simulink model "vanderpol_simulink"  (R2013a)
settings: Solver=ode45  StartTime=0.0  StopTime=2  RelTol=1e-3
settings Model: Creator=zutshi  LastModifiedBy=zutshi

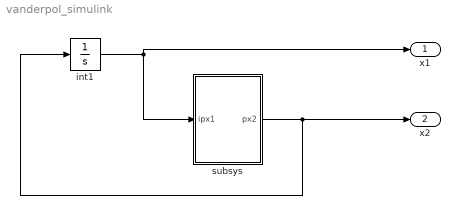
== system vanderpol_simulink ==
  int1 : Integrator  InitialCondition=0.4611  ContinuousStateAttributes='x1'
  subsys : Subsystem
  x1 : Outport
  x2 : Outport  Port=2
  wires:
  int1/1 -> x1/1, subsys/1(ipx1)
  subsys/1(px2) -> x2/1, int1/1

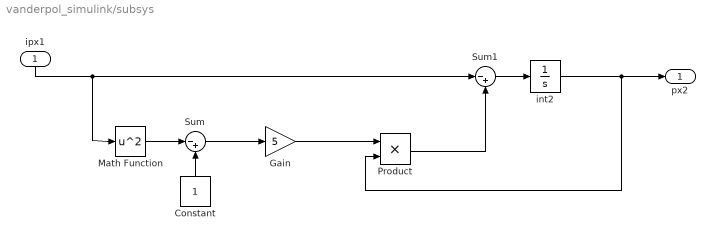
== system vanderpol_simulink/subsys ==
  ipx1 : Inport
  Constant : Constant
  Gain : Gain  Gain=5
  Math Function : Math  Operator=square  SaturateOnIntegerOverflow=on
  Product : Product
  Sum : Sum  Inputs=|-+
  Sum1 : Sum  Inputs=|-+
  int2 : Integrator  InitialCondition=-0.40808  ContinuousStateAttributes='x2'
  px2 : Outport
  wires:
  ipx1/1 -> Sum1/1, Math Function/1
  Constant/1 -> Sum/2
  Sum1/1 -> int2/1
  int2/1 -> Product/2, px2/1
  Sum/1 -> Gain/1
  Product/1 -> Sum1/2
  Math Function/1 -> Sum/1
  Gain/1 -> Product/1
